simulink model "AMCLIB_Windmilling_BAM"  (Simulink 9.3)
settings: Solver=VariableStepAuto  StartTime=0.0  StopTime=10.0  RelTol=1e-3
settings Model: Creator=nxa18952  LastModifiedBy=nxa18952
settings DataIOCC: SaveFormat=Dataset  SignalLoggingSaveFormat=Dataset  ReturnWorkspaceOutputs=on
settings OptimizationCC: LifeSpan=auto
settings DebuggingCC: UnderspecifiedInitializationDetection=Simplified  MergeDetectMultiDrivingBlocksExec=error  FcnCallInpInsideContextMsg=error  SFUnexpectedBacktrackingDiag=error  SFNoUnconditionalDefaultTransitionDiag=error  SFExecutionAtInitializationDiag=warning  ArithmeticOperatorsInVariantConditions=error
settings HardwareCC: ProdBitPerPointer=64  ProdBitPerSizeT=64  ProdBitPerPtrDiffT=64  ProdLargestAtomicFloat=Float  ProdIntDivRoundTo=Zero  ProdEndianess=LittleEndian  ProdWordSize=64  ProdHWDeviceType=Intel->x86-64 (Windows64)
settings ModelReferenceCC: PropagateSignalLabelsOutOfModel=on
settings SFSimCC: SimUseLocalCustomCode=on
settings RTWCC: RTWUseLocalCustomCode=on
settings CodeAppCC: StateflowObjectComments=off
settings GRTTargetCC: TargetLangStandard=C99 (ISO)  CombineOutputUpdateFcns=on  GRTInterface=off
settings ConfigComp: CovMetricSettings=dwe  CovHtmlReporting=off  CovSaveCumulativeToWorkspaceVar=off  CovSaveSingleToWorkspaceVar=off  CovExternalEMLEnable=on

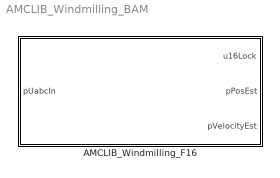
== system AMCLIB_Windmilling_BAM ==
  AMCLIB_Windmilling_F16 : Subsystem  TreatAsAtomicUnit=on  mask(AMCLIB_Windmilling_F16){showStates=Hide (faster execution), f16ADCMaxError=0, f16CC1sc=0, f16CC2sc=0, f16UpperLimit=0, f16LowerLimit=0, u16NShiftPI=0, f16C1=0, u16NShiftI=0}
      mask prompts: showStates "Show internal states"; f16ADCMaxError "f16ADCMaxError (Maximum differential offset error between any two phases of the 3-phase voltage-sensing A/D converters.)"; f16CC1sc "f16CC1sc (GFLIB_ControllerPIrAW - CC1 coefficient)"; f16CC2sc "f16CC2sc (GFLIB_ControllerPIrAW - CC2 coefficient)"; f16UpperLimit "f16UpperLimit (GFLIB_ControllerPIrAW - upper Limit of the controller)"; f16LowerLimit "f16LowerLimit (GFLIB_ControllerPIrAW - lower Limit of the controller)"; u16NShiftPI "u16NShiftPI (GFLIB_ControllerPIrAW - scaling bitwise shift applied to the controller coefficients)"; f16C1 "f16C1 (GFLIB_IntegratorTR - integrator coefficient)"; u16NShiftI "u16NShiftI (GFLIB_IntegratorTR - scaling bitwise shift applied to the integrator coefficient)"
      mask help: PMSM Windmilling in 16-bit fixed-point fractional implementation. This function detects spontaneous rotation of an unpowered 3-phase PMSM by measuring the generated back electromotive force. Output u16Lock represents the return value of the C function (0 = undecided, 1 = spinning, 2 = stopped). Transition from 0 to 1 on the u16Lock output can be taken as a reset signal for the following AMCLIB_TrackObsrv_F16 block to synchronize the sensorless FOC loop with a freewheeling motor. Refer to the AMMCLIB User's Guide for further details.
      mask init:
      | if ~evalin('base','exist(''tS8'',''var'')')
      |   if (2 ~= exist('SWLIBS_Typedefs.mat','file'))
      |       error('File SWLIBS_Typedefs.mat is not on the Matlab path. Please add the AMMCLIB "bam" folder in the Matlab Search Path.');
      |   else
      |       evalin('base', 'load(''SWLIBS_Typedefs.mat'')');
      |   end
      | end
      | if showStates == 1
      |     % hidden state variables
      |     if strcmp(get_param([gcb '/f16ADCMaxError'], 'BlockType'), 'Inport')
      |         posblk = get_param(gcb, 'Position');
      | 
      |         pos = get_param(    [gcb, '/f16ADCMaxError'], 'Position');
      |         orient = get_param( [gcb, '/f16ADCMaxError'], 'Orientation');
      |         delete_block(       [gcb, '/f16ADCMaxError']);
      |         add_block('built-in/Ground', [gcb, '/f16ADCMaxError'], 'Position', pos, 'Orientation', orient);
      | 
      |         pos = get_param(    [gcb, '/f16CC1sc'], 'Position');
      |         orient = get_param( [gcb, '/f16CC1sc'], 'Orientation');
      |         delete_block(       [gcb, '/f16CC1sc']);
      |         add_block('built-in/Ground', [gcb, '/f16CC1sc'], 'Position', pos, 'Orientation', orient);
      | 
      |         pos = get_param(    [gcb, '/f16CC2sc'], 'Position');
      |         orient = get_param( [gcb, '/f16CC2sc'], 'Orientation');
      |         delete_block(       [gcb, '/f16CC2sc']);
      |         add_block('built-in/Ground', [gcb, '/f16CC2sc'], 'Position', pos, 'Orientation', orient);
      | 
      |         pos = get_param(    [gcb, '/f16UpperLimit'], 'Position');
      |         orient = get_param( [gcb, '/f16UpperLimit'], 'Orientation');
      |         delete_block(       [gcb, '/f16UpperLimit']);
      |         add_block('built-in/Ground', [gcb, '/f16UpperLimit'], 'Position', pos, 'Orientation', orient);
      | 
      |         pos = get_param(    [gcb, '/f16LowerLimit'], 'Position');
      |         orient = get_param( [gcb, '/f16LowerLimit'], 'Orientation');
      |         delete_block(       [gcb, '/f16LowerLimit']);
      |         add_block('built-in/Ground', [gcb, '/f16LowerLimit'], 'Position', pos, 'Orientation', orient);
      | 
      |         pos = get_param(    [gcb, '/u16NShiftPI'], 'Position');
      |         orient = get_param( [gcb, '/u16NShiftPI'], 'Orientation');
      |         delete_block(       [gcb, '/u16NShiftPI']);
      |         add_block('built-in/Ground', [gcb, '/u16NShiftPI'], 'Position', pos, 'Orientation', orient);
      | 
      |         pos = get_param(    [gcb, '/f16C1'], 'Position');
      |         orient = get_param( [gcb, '/f16C1'], 'Orientation');
      |         delete_block(       [gcb, '/f16C1']);
      |         add_block('built-in/Ground', [gcb, '/f16C1'], 'Position', pos, 'Orientation', orient);
      | 
      |         pos = get_param(    [gcb, '/u16NShiftI'], 'Position');
      |         orient = get_param( [gcb, '/u16NShiftI'], 'Orientation');
      |         delete_block(       [gcb, '/u16NShiftI']);
      |         add_block('built-in/Ground', [gcb, '/u16NShiftI'], 'Position', pos, 'Orientation', orient);
      | 
      |         pos = get_param(    [gcb, '/f32AccPI'], 'Position');
      |         orient = get_param( [gcb, '/f32AccPI'], 'Orientation');
      |         delete_block(       [gcb, '/f32AccPI']);
      |         add_block('built-in/Ground', [gcb, '/f32AccPI'], 'Position', pos, 'Orientation', orient);
      | 
      |         pos = get_param(    [gcb, '/f16InErrK1'], 'Position');
      |         orient = get_param( [gcb, '/f16InErrK1'], 'Orientation');
      |         delete_block(       [gcb, '/f16InErrK1']);
      |         add_block('built-in/Ground', [gcb, '/f16InErrK1'], 'Position', pos, 'Orientation', orient);
      | 
      |         pos = get_param(    [gcb, '/f32State'], 'Position');
      |         orient = get_param( [gcb, '/f32State'], 'Orientation');
      |         delete_block(       [gcb, '/f32State']);
      |         add_block('built-in/Ground', [gcb, '/f32State'], 'Position', pos, 'Orientation', orient);
      | 
      |         pos = get_param(    [gcb, '/f16InK1'], 'Position');
      |         orient = get_param( [gcb, '/f16InK1'], 'Orientation');
      |         delete_block(       [gcb, '/f16InK1']);
      |         add_block('built-in/Ground', [gcb, '/f16InK1'], 'Position', pos, 'Orientation', orient);
      | 
      | 
      |         pos = get_param(    [gcb '/f32AccPI_Out'], 'Position');
      |         orient = get_param( [gcb '/f32AccPI_Out'], 'Orientation');
      |         delete_block(       [gcb '/f32AccPI_Out']);
      |         add_block('built-in/Terminator', [gcb '/f32AccPI_Out'], 'Position', pos, 'Orientation', orient);
      | 
      |         pos = get_param(    [gcb '/f16InErrK1_Out'], 'Position');
      |         orient = get_param( [gcb '/f16InErrK1_Out'], 'Orientation');
      |         delete_block(       [gcb '/f16InErrK1_Out']);
      |         add_block('built-in/Terminator', [gcb '/f16InErrK1_Out'], 'Position', pos, 'Orientation', orient);
      | 
      |         pos = get_param(    [gcb '/f32State_Out'], 'Position');
      |         orient = get_param( [gcb '/f32State_Out'], 'Orientation');
      |         delete_block(       [gcb '/f32State_Out']);
      |         add_block('built-in/Terminator', [gcb '/f32State_Out'], 'Position', pos, 'Orientation', orient);
      | 
      |         pos = get_param(    [gcb '/f16InK1_Out'], 'Position');
      |         orient = get_param( [gcb '/f16InK1_Out'], 'Orientation');
      |         delete_block(       [gcb '/f16InK1_Out']);
      |         add_block('built-in/Terminator', [gcb '/f16InK1_Out'], 'Position', pos, 'Orientation', orient);
      | 
      | 
      |         set_param([gcb '/pUabcIn'], 'Port', '1');
      | 
      |         set_param([gcb '/u16Lock'], 'Port', '1');
      |         set_param([gcb '/pPosEst'], 'Port', '2');
      |         set_param([gcb '/pVelocityEst'], 'Port', '3');
      | 
      |         set_param(gcb,'MaskEnables',{'on','on','on','on','on','on','on','on','on'});
      | 
      |         if (posblk(4) - posblk(2)) > 100
      |           height = 100;
      |           set_param(gcb,'Position',[posblk(1), posblk(2), posblk(3), posblk(2)+height])
      |         end
      |     end
      | else
      |     % shown state variables
      |     if strcmp(get_param([gcb '/f16ADCMaxError'], 'BlockType'), 'Ground')
      |         posblk = get_param(gcb, 'Position');
      | 
      |         pos = get_param(    [gcb, '/f16ADCMaxError'], 'Position');
      |         orient = get_param( [gcb, '/f16ADCMaxError'], 'Orientation');
      |         delete_block(       [gcb, '/f16ADCMaxError']);
      |         add_block('built-in/Inport', [gcb, '/f16ADCMaxError'], 'Position', pos, 'Orientation', orient, 'OutDataTypeStr', 'int16');
      | 
      |         pos = get_param(    [gcb, '/f16CC1sc'], 'Position');
      |         orient = get_param( [gcb, '/f16CC1sc'], 'Orientation');
      |         delete_block(       [gcb, '/f16CC1sc']);
      |         add_block('built-in/Inport', [gcb, '/f16CC1sc'], 'Position', pos, 'Orientation', orient, 'OutDataTypeStr', 'int16');
      | 
      |         pos = get_param(    [gcb, '/f16CC2sc'], 'Position');
      |         orient = get_param( [gcb, '/f16CC2sc'], 'Orientation');
      |         delete_block(       [gcb, '/f16CC2sc']);
      |         add_block('built-in/Inport', [gcb, '/f16CC2sc'], 'Position', pos, 'Orientation', orient, 'OutDataTypeStr', 'int16');
      | 
      |         pos = get_param(    [gcb, '/f16UpperLimit'], 'Position');
      |         orient = get_param( [gcb, '/f16UpperLimit'], 'Orientation');
      |         delete_block(       [gcb, '/f16UpperLimit']);
      |         add_block('built-in/Inport', [gcb, '/f16UpperLimit'], 'Position', pos, 'Orientation', orient, 'OutDataTypeStr', 'int16');
      | 
      |         pos = get_param(    [gcb, '/f16LowerLimit'], 'Position');
      |         orient = get_param( [gcb, '/f16LowerLimit'], 'Orientation');
      |         delete_block(       [gcb, '/f16LowerLimit']);
      |         add_block('built-in/Inport', [gcb, '/f16LowerLimit'], 'Position', pos, 'Orientation', orient, 'OutDataTypeStr', 'int16');
      | 
      |         pos = get_param(    [gcb, '/u16NShiftPI'], 'Position');
      |         orient = get_param( [gcb, '/u16NShiftPI'], 'Orientation');
      |         delete_block(       [gcb, '/u16NShiftPI']);
      |         add_block('built-in/Inport', [gcb, '/u16NShiftPI'], 'Position', pos, 'Orientation', orient, 'OutDataTypeStr', 'uint16');
      | 
      |         pos = get_param(    [gcb, '/f16C1'], 'Position');
      |         orient = get_param( [gcb, '/f16C1'], 'Orientation');
      |         delete_block(       [gcb, '/f16C1']);
      |         add_block('built-in/Inport', [gcb, '/f16C1'], 'Position', pos, 'Orientation', orient, 'OutDataTypeStr', 'int16');
      | 
      |         pos = get_param(    [gcb, '/u16NShiftI'], 'Position');
      |         orient = get_param( [gcb, '/u16NShiftI'], 'Orientation');
      |         delete_block(       [gcb, '/u16NShiftI']);
      |         add_block('built-in/Inport', [gcb, '/u16NShiftI'], 'Position', pos, 'Orientation', orient, 'OutDataTypeStr', 'uint16');
      | 
      |         pos = get_param(    [gcb, '/f32AccPI'], 'Position');
      |         orient = get_param( [gcb, '/f32AccPI'], 'Orientation');
      |         delete_block(       [gcb, '/f32AccPI']);
      |         add_block('built-in/Inport', [gcb, '/f32AccPI'], 'Position', pos, 'Orientation', orient, 'OutDataTypeStr', 'int32');
      | 
      |         pos = get_param(    [gcb, '/f16InErrK1'], 'Position');
      |         orient = get_param( [gcb, '/f16InErrK1'], 'Orientation');
      |         delete_block(       [gcb, '/f16InErrK1']);
      |         add_block('built-in/Inport', [gcb, '/f16InErrK1'], 'Position', pos, 'Orientation', orient, 'OutDataTypeStr', 'int16');
      | 
      |         pos = get_param(    [gcb, '/f32State'], 'Position');
      |         orient = get_param( [gcb, '/f32State'], 'Orientation');
      |         delete_block(       [gcb, '/f32State']);
      |         add_block('built-in/Inport', [gcb, '/f32State'], 'Position', pos, 'Orientation', orient, 'OutDataTypeStr', 'int32');
      | 
      |         pos = get_param(    [gcb, '/f16InK1'], 'Position');
      |         orient = get_param( [gcb, '/f16InK1'], 'Orientation');
      |         delete_block(       [gcb, '/f16InK1']);
      |         add_block('built-in/Inport', [gcb, '/f16InK1'], 'Position', pos, 'Orientation', orient, 'OutDataTypeStr', 'int16');
      | 
      | 
      |         pos = get_param(    [gcb '/f32AccPI_Out'], 'Position');
      |         orient = get_param( [gcb '/f32AccPI_Out'], 'Orientation');
      |         delete_block(       [gcb '/f32AccPI_Out']);
      |         add_block('built-in/Outport', [gcb '/f32AccPI_Out'], 'Position', pos, 'Orientation', orient);
      | 
      |         pos = get_param(    [gcb '/f16InErrK1_Out'], 'Position');
      |         orient = get_param( [gcb '/f16InErrK1_Out'], 'Orientation');
      |         delete_block(       [gcb '/f16InErrK1_Out']);
      |         add_block('built-in/Outport', [gcb '/f16InErrK1_Out'], 'Position', pos, 'Orientation', orient);
      | 
      |         pos = get_param(    [gcb '/f32State_Out'], 'Position');
      |         orient = get_param( [gcb '/f32State_Out'], 'Orientation');
      |         delete_block(       [gcb '/f32State_Out']);
      |         add_block('built-in/Outport', [gcb '/f32State_Out'], 'Position', pos, 'Orientation', orient);
      | 
      |         pos = get_param(    [gcb '/f16InK1_Out'], 'Position');
      |         orient = get_param( [gcb '/f16InK1_Out'], 'Orientation');
      |         delete_block(       [gcb '/f16InK1_Out']);
      |         add_block('built-in/Outport', [gcb '/f16InK1_Out'], 'Position', pos, 'Orientation', orient);
      | 
      | 
      |         set_param([gcb '/pUabcIn'], 'Port', '1');
      |         set_param([gcb '/f16ADCMaxError'], 'Port', '2');
      |         set_param([gcb '/f16CC1sc'], 'Port', '3');
      |         set_param([gcb '/f16CC2sc'], 'Port', '4');
      |         set_param([gcb '/f16UpperLimit'], 'Port', '5');
      |         set_param([gcb '/f16LowerLimit'], 'Port', '6');
      |         set_param([gcb '/u16NShiftPI'], 'Port', '7');
      |         set_param([gcb '/f16C1'], 'Port', '8');
      |         set_param([gcb '/u16NShiftI'], 'Port', '9');
      |         set_param([gcb '/f32AccPI'], 'Port', '10');
      |         set_param([gcb '/f16InErrK1'], 'Port', '11');
      |         set_param([gcb '/f32State'], 'Port', '12');
      |         set_param([gcb '/f16InK1'], 'Port', '13');
      | 
      |         set_param([gcb '/u16Lock'], 'Port', '1');
      |         set_param([gcb '/pPosEst'], 'Port', '2');
      |         set_param([gcb '/pVelocityEst'], 'Port', '3');
      |         set_param([gcb '/f32AccPI_Out'], 'Port', '4');
      |         set_param([gcb '/f16InErrK1_Out'], 'Port', '5');
      |         set_param([gcb '/f32State_Out'], 'Port', '6');
      |         set_param([gcb '/f16InK1_Out'], 'Port', '7');
      | 
      |         set_param(gcb,'MaskEnables',{'on','off','off','off','off','off','off','off','off'});
      | 
      |         if (posblk(4) - posblk(2)) < 350
      |           height = 350;
      |           set_param(gcb,'Position',[posblk(1), posblk(2), posblk(3), posblk(2)+height])
      |         end
      |     end
      | end
      settings: RTWSystemCode=Inline
      mask TypeOptions showStates: Hide (faster execution) | Show (allows debugging; connect feedback loops manually)
      mask Callback showStates:
      | maskStr = get_param(gcb,'showStates');
      | if strcmp(maskStr,'Hide (faster execution)'),
      |     set_param(gcb,'MaskEnables',{'on','on','on','on','on','on','on','on','on'});
      | else
      |     set_param(gcb,'MaskEnables',{'on','off','off','off','off','off','off','off','off'});
      | end
      mask Display:
      | color('black');
      | pos = get_param(gcb, 'Position');
      | width = pos(3) - pos(1);
      | height = pos(4) - pos(2);
      | tX=width/2;
      | tY=height - 8;
      | color('black');
      | text(tX,tY, 'AMCLIB_Windmilling_F16', 'horizontalAlignment', 'center');
      | if showStates == 2
      |   color('red');
      |   text(tX,tY - 20, ['debugging mode' char(13) char(10) '(limited performance)'], 'horizontalAlignment', 'center');
      | end

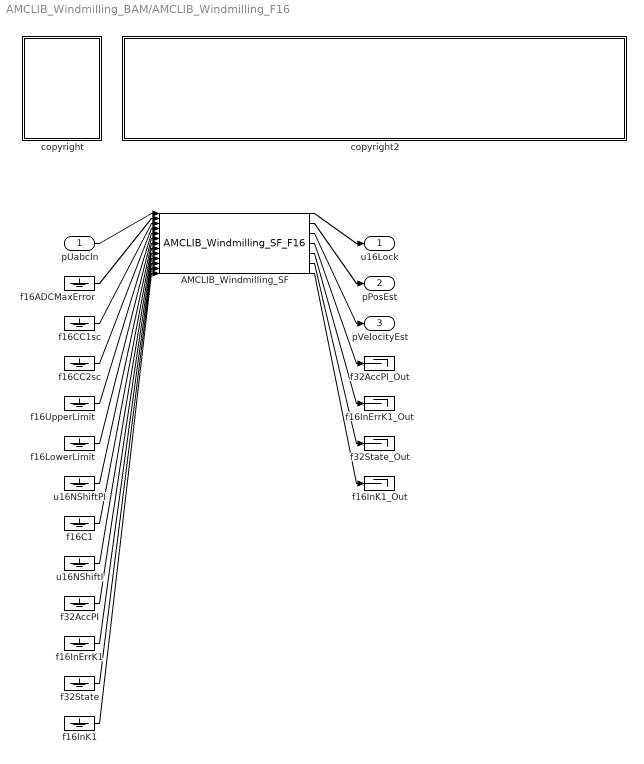
== system AMCLIB_Windmilling_BAM/AMCLIB_Windmilling_F16 ==
  pUabcIn : Inport  OutDataTypeStr=Bus: SWLIBS_3Syst_F16  BusOutputAsStruct=on
  AMCLIB_Windmilling_SF : S-Function  FunctionName=AMCLIB_Windmilling_SF_F16  Parameters=showStates,f16ADCMaxError,f16CC1sc,f16CC2sc,f16UpperLimit,f16LowerLimit,u16NShiftPI,f16C1,u16NShiftI  SFunctionDeploymentMode=off  EnableBusSupport=off
  copyright : Subsystem
      mask Display: text(10,90,'FILE:');text(10,75,'DESRIPTION:');text(10,60,'COPYRIGHT:');text(10,45,'VERSION:');text(10,30,'DATE:')
  copyright2 : Subsystem
      mask Display: text(10,90,'AMCLIB_Windmilling_BAM_F16.mdl');text(10,75,'PMSM Windmilling');text(10,60,'NXP 2020');text(10,45,'1.0');text(10,30,'28-Mar-2020');
  f16ADCMaxError : Ground
  f16C1 : Ground
  f16CC1sc : Ground
  f16CC2sc : Ground
  f16InErrK1 : Ground
  f16InErrK1_Out : Terminator
  f16InK1 : Ground
  f16InK1_Out : Terminator
  f16LowerLimit : Ground
  f16UpperLimit : Ground
  f32AccPI : Ground
  f32AccPI_Out : Terminator
  f32State : Ground
  f32State_Out : Terminator
  u16NShiftI : Ground
  u16NShiftPI : Ground
  u16Lock : Outport
  pPosEst : Outport  Port=2
  pVelocityEst : Outport  Port=3
  wires:
  pUabcIn/1 -> AMCLIB_Windmilling_SF/1
  f16ADCMaxError/1 -> AMCLIB_Windmilling_SF/2
  f16CC1sc/1 -> AMCLIB_Windmilling_SF/3
  f16CC2sc/1 -> AMCLIB_Windmilling_SF/4
  f16UpperLimit/1 -> AMCLIB_Windmilling_SF/5
  f16LowerLimit/1 -> AMCLIB_Windmilling_SF/6
  u16NShiftPI/1 -> AMCLIB_Windmilling_SF/7
  f16C1/1 -> AMCLIB_Windmilling_SF/8
  u16NShiftI/1 -> AMCLIB_Windmilling_SF/9
  f32AccPI/1 -> AMCLIB_Windmilling_SF/10
  f16InErrK1/1 -> AMCLIB_Windmilling_SF/11
  f32State/1 -> AMCLIB_Windmilling_SF/12
  f16InK1/1 -> AMCLIB_Windmilling_SF/13
  AMCLIB_Windmilling_SF/1 -> u16Lock/1
  AMCLIB_Windmilling_SF/2 -> pPosEst/1
  AMCLIB_Windmilling_SF/3 -> pVelocityEst/1
  AMCLIB_Windmilling_SF/4 -> f32AccPI_Out/1
  AMCLIB_Windmilling_SF/5 -> f16InErrK1_Out/1
  AMCLIB_Windmilling_SF/6 -> f32State_Out/1
  AMCLIB_Windmilling_SF/7 -> f16InK1_Out/1

== system AMCLIB_Windmilling_BAM/AMCLIB_Windmilling_F16/copyright ==

== system AMCLIB_Windmilling_BAM/AMCLIB_Windmilling_F16/copyright2 ==
